simulink model "IFSSIM_Brakes"  (R2025b)
settings: Solver=FixedStepDiscrete  StartTime=0  StopTime=inf  FixedStep=1/960  RelTol=1e-3
undefined symbols (not defined in the file or in its folder): IFSSIM_ebstau, IFSSIM_Tebs, IFSSIM_Ts
settings Model: Creator=raulmoran  LastModifiedBy=raulmoran

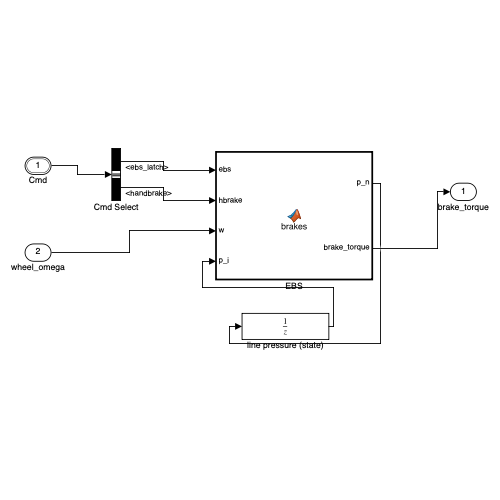
[thumbnail: Simulink's stored preview of the top-level diagram]
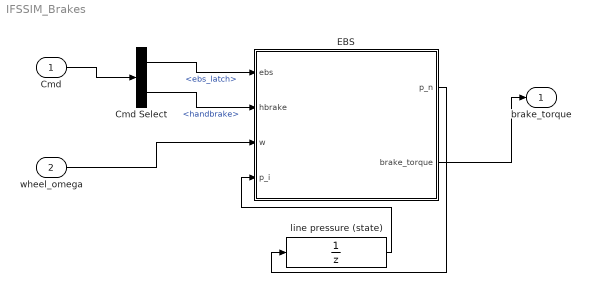
== system IFSSIM_Brakes ==
  Cmd : Inport  OutDataTypeStr=Bus: IFSSIM_CmdBus  BusOutputAsStruct=on
  wheel_omega : Inport  Port=2  PortDimensions=4
  Cmd Select : BusSelector  OutputSignals=ebs_latch,handbrake
  EBS : MATLAB Function  TreatAsAtomicUnit=on
  line pressure (state) : UnitDelay  SampleTime=-1  HasFrameUpgradeWarning=on
  brake_torque : Outport  PortDimensions=4
  wires:
  Cmd/1 -> Cmd Select/1
  Cmd Select/1 -> EBS/1(ebs)  "<ebs_latch>"
  Cmd Select/2 -> EBS/2(hbrake)  "<handbrake>"
  wheel_omega/1 -> EBS/3(w)
  line pressure (state)/1 -> EBS/4(p_i)
  EBS/1(p_n) -> line pressure (state)/1
  EBS/2(brake_torque) -> brake_torque/1

== matlab function IFSSIM_Brakes/EBS ==
  data: ebs input size=1; p_n output size=1; hbrake input size=1; w input size=4; p_i input size=1; brake_torque output size=4; IFSSIM_Ts parameter size=1; IFSSIM_Tebs parameter size=1; IFSSIM_ebstau parameter size=1
function [p_n, brake_torque] = brakes(ebs, hbrake, w, p_i, IFSSIM_Ts, IFSSIM_Tebs, IFSSIM_ebstau)
%#codegen
% EBS only. There is no hydraulic service brake on this car; regen does that
% job and arrives at the tyre as negative drive torque from the powertrain.

Ts = IFSSIM_Ts;

% Either channel commands the same pneumatic system. They are separate inputs
% because the LATCH logic differs upstream — EBS latches until the mission
% flow releases it, the handbrake does not — but the hardware is one system.
demand = max(ebs, hbrake);
demand = max(0, min(1, demand));

% Line pressure as a first-order fill. Defaulted to effectively instant, so
% this is a hook rather than a model until someone measures the real system.
alpha = min(Ts / max(IFSSIM_ebstau, 1e-9), 1);
p_n = p_i + alpha * (demand - p_i);

% Magnitude only. The tyre block owns the sign, because it owns the wheel
% state and is the only place that knows which way the wheel is turning.
T = p_i * IFSSIM_Tebs;
brake_torque = [T; T; T; T];
end
